simulink model "L3Pilot_AEB_v1"  (R2021b)
settings: Solver=FixedStepAuto  StartTime=0.0  StopTime=350  RelTol=1e-3  EnableMultiTasking=on
values from neighbouring files (symbols this model uses):
  t_takeover = 70    [Var_L3Pilot_ADF_v1.m]
  Tabt = 0.1    [Var_L3Pilot_ADF_v1.m]
undefined symbols (not defined in the file or in its folder): ComponentState
libraries: simulink x2
settings Model: Creator=QXV8396  LastModifiedBy=Q395473
settings SolverCC: AlgebraicLoopSolver=TrustRegion
settings DataIOCC: LimitDataPoints=on  ReturnWorkspaceOutputs=off
settings DebuggingCC: AllowSymbolicDim=off  SFUnexpectedBacktrackingDiag=warning  SFNoUnconditionalDefaultTransitionDiag=warning  SFExecutionAtInitializationDiag=none  SFMachineParentedDataDiag=warning  ArithmeticOperatorsInVariantConditions=warning
settings ModelReferenceCC: PropagateSignalLabelsOutOfModel=off
settings SFSimCC: SimUseLocalCustomCode=off  CustomCodeUndefinedFunction=UseInterfaceOnly
settings RTWCC: Description=FMU Co-Simulation 1.0 Standalone  SystemTargetFile=fmu_cs1.tlc  MakeCommand=make_rtw FMIT_INTERMEDIATE_LIB_DIR=DEFAULT FMIT_ADDITIONAL_CFLAGS=  TemplateMakefile=fmu_cs1_default_tmf  RTWUseLocalCustomCode=off
settings CodeAppCC: StateflowObjectComments=on
settings STFCustomTargetCC: MATLABClassNameForMDSCustomization=Simulink.SoftwareTarget.TargetSpecificTriggerConfigurationBase  SystemTargetFile=fmu_cs1.tlc
settings ConfigComp: CovMetricSettings=dw  CovSaveCumulativeToWorkspaceVar=on  CovSaveSingleToWorkspaceVar=on  CovExternalEMLEnable=off

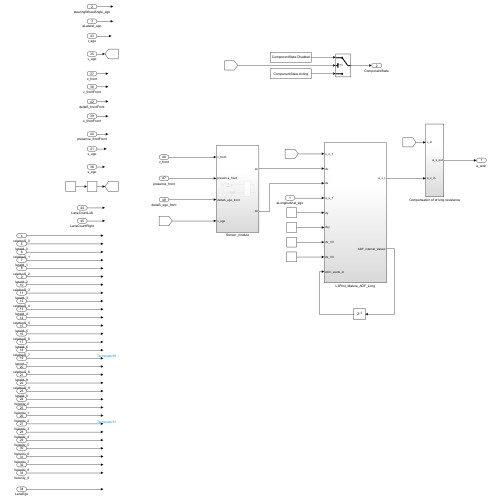
[thumbnail: Simulink's stored preview of the top-level diagram]
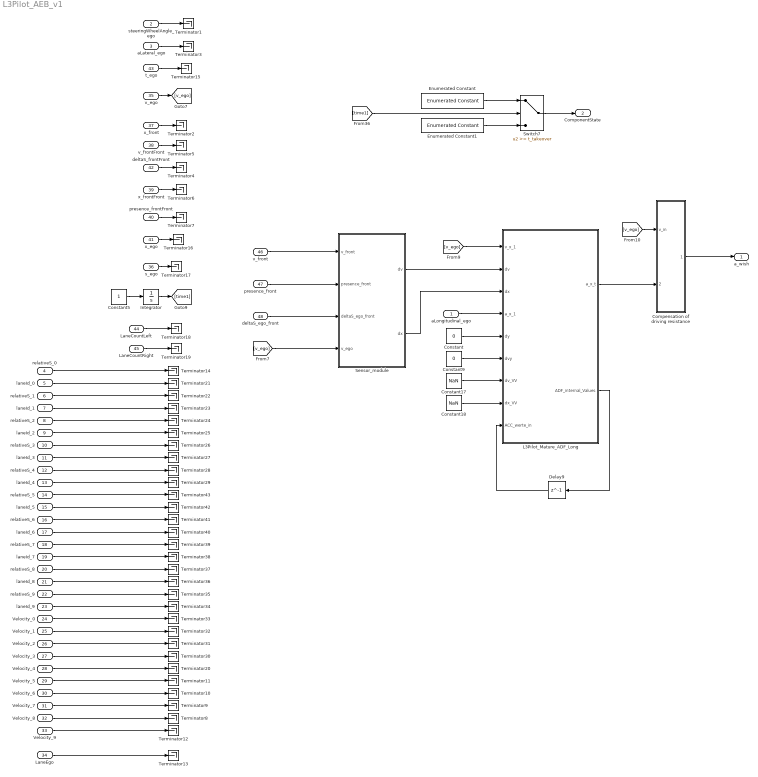
== system L3Pilot_AEB_v1 ==
  aLongitudinal_ego : Inport
  steeringWheelAngle_ego : Inport  Port=2
  aLateral_ego : Inport  Port=3
  relativeS_0 : Inport  Port=4  OutDataTypeStr=double
  laneId_0 : Inport  Port=5  OutDataTypeStr=int8
  relativeS_1 : Inport  Port=6  OutDataTypeStr=double
  laneId_1 : Inport  Port=7  OutDataTypeStr=int8
  relativeS_2 : Inport  Port=8  OutDataTypeStr=double
  laneId_2 : Inport  Port=9  OutDataTypeStr=int8
  relativeS_3 : Inport  Port=10  OutDataTypeStr=double
  laneId_3 : Inport  Port=11  OutDataTypeStr=int8
  relativeS_4 : Inport  Port=12  OutDataTypeStr=double
  laneId_4 : Inport  Port=13  OutDataTypeStr=int8
  relativeS_5 : Inport  Port=14  OutDataTypeStr=double
  laneId_5 : Inport  Port=15  OutDataTypeStr=int8
  relativeS_6 : Inport  Port=16  OutDataTypeStr=double
  laneId_6 : Inport  Port=17  OutDataTypeStr=int8
  relativeS_7 : Inport  Port=18  OutDataTypeStr=double
  laneId_7 : Inport  Port=19  OutDataTypeStr=int8
  relativeS_8 : Inport  Port=20  OutDataTypeStr=double
  laneId_8 : Inport  Port=21  OutDataTypeStr=int8
  relativeS_9 : Inport  Port=22  OutDataTypeStr=double
  laneId_9 : Inport  Port=23  OutDataTypeStr=int8
  Velocity_0 : Inport  Port=24  OutDataTypeStr=double
  Velocity_1 : Inport  Port=25  OutDataTypeStr=double
  Velocity_2 : Inport  Port=26  OutDataTypeStr=double
  Velocity_3 : Inport  Port=27  OutDataTypeStr=double
  Velocity_4 : Inport  Port=28  OutDataTypeStr=double
  Velocity_5 : Inport  Port=29  OutDataTypeStr=double
  Velocity_6 : Inport  Port=30  OutDataTypeStr=double
  Velocity_7 : Inport  Port=31  OutDataTypeStr=double
  Velocity_8 : Inport  Port=32  OutDataTypeStr=double
  Velocity_9 : Inport  Port=33  OutDataTypeStr=double
  LaneEgo : Inport  Port=34  OutDataTypeStr=int8
  v_ego : Inport  Port=35  OutDataTypeStr=double
  s_ego : Inport  Port=36
  x_front : Inport  Port=37  OutDataTypeStr=double
  v_frontFront : Inport  Port=38  OutDataTypeStr=double
  x_frontFront : Inport  Port=39  OutDataTypeStr=double
  presence_frontFront : Inport  Port=40  OutDataTypeStr=boolean
  x_ego : Inport  Port=41
  deltaS_frontFront : Inport  Port=42  OutDataTypeStr=double
  t_ego : Inport  Port=43
  LaneCountLeft : Inport  Port=44  OutDataTypeStr=int8
  LaneCountRight : Inport  Port=45  OutDataTypeStr=int8
  v_front : Inport  Port=46  OutDataTypeStr=double
  presence_front : Inport  Port=47  OutDataTypeStr=boolean
  deltaS_ego_front : Inport  Port=48
  Compensation of driving resistance : Subsystem
  Constant : Constant  Value=0  SampleTime=Tabt
  Constant17 : Constant  Value=NaN  SampleTime=Tabt
  Constant18 : Constant  Value=NaN  SampleTime=Tabt
  Constant5 : Constant  SampleTime=Tabt
  Constant9 : Constant  Value=0  SampleTime=Tabt
  Delay9 : Delay  DelayLength=1  InitialCondition=0  SampleTime=Tabt
  Enumerated Constant : simulink/Sources/Enumerated Constant  OutDataTypeStr=Enum: ComponentState  Value=ComponentState.Disabled  SampleTime=inf
  Enumerated Constant1 : simulink/Sources/Enumerated Constant  OutDataTypeStr=Enum: ComponentState  Value=ComponentState.Acting  SampleTime=inf
  Integrator : Integrator
  L3Pilot_Mature_ADF_Long : Subsystem
  Sensor_module : Subsystem
  Switch7 : Switch  Threshold=t_takeover
  Terminator{1..43} (43 alike) : Terminator
  a_wish : Outport  VectorParamsAs1DForOutWhenUnconnected=off
  ComponentState : Outport  Port=2  OutDataTypeStr=Enum: ComponentState  VectorParamsAs1DForOutWhenUnconnected=off
  wires:
  Constant17/1 -> L3Pilot_Mature_ADF_Long/7(dv_VV)
  Constant18/1 -> L3Pilot_Mature_ADF_Long/8(dx_VV)
  Constant9/1 -> L3Pilot_Mature_ADF_Long/6(dvy)
  Constant/1 -> L3Pilot_Mature_ADF_Long/5(dy)
  Delay9/1 -> L3Pilot_Mature_ADF_Long/9(ACC_werte_in)
  aLongitudinal_ego/1 -> L3Pilot_Mature_ADF_Long/4("a_x_1 ")
  L3Pilot_Mature_ADF_Long/2(ADF_internal_Values) -> Delay9/1
  [v_ego] -> L3Pilot_Mature_ADF_Long/1(v_x_1)
  [v_ego] -> Compensation of driving resistance/1(v_in)
  Sensor_module/1(dv) -> L3Pilot_Mature_ADF_Long/2(dv)
  Sensor_module/2(dx) -> L3Pilot_Mature_ADF_Long/3(dx)
  L3Pilot_Mature_ADF_Long/1(a_x_t) -> Compensation of driving resistance/2(a_x_in)
  Compensation of driving resistance/1(a_x_out) -> a_wish/1
  relativeS_1/1 -> Terminator22/1
  Velocity_2/1 -> Terminator31/1
  laneId_9/1 -> Terminator34/1
  relativeS_4/1 -> Terminator28/1
  [time1] -> Switch7/2
  Velocity_4/1 -> Terminator20/1
  Switch7/1 -> ComponentState/1
  Velocity_8/1 -> Terminator8/1
  Velocity_9/1 -> Terminator12/1
  relativeS_8/1 -> Terminator37/1
  relativeS_2/1 -> Terminator24/1
  relativeS_9/1 -> Terminator35/1
  Velocity_1/1 -> Terminator32/1
  relativeS_7/1 -> Terminator39/1
  relativeS_6/1 -> Terminator41/1
  relativeS_0/1 -> Terminator14/1
  laneId_7/1 -> Terminator38/1
  relativeS_5/1 -> Terminator43/1
  laneId_2/1 -> Terminator25/1
  laneId_3/1 -> Terminator27/1
  laneId_1/1 -> Terminator23/1
  Velocity_3/1 -> Terminator30/1
  Velocity_6/1 -> Terminator10/1
  LaneEgo/1 -> Terminator13/1
  Velocity_7/1 -> Terminator9/1
  Velocity_5/1 -> Terminator11/1
  relativeS_3/1 -> Terminator26/1
  laneId_6/1 -> Terminator40/1
  laneId_8/1 -> Terminator36/1
  laneId_4/1 -> Terminator29/1
  Enumerated Constant1/1 -> Switch7/3
  Enumerated Constant/1 -> Switch7/1
  laneId_5/1 -> Terminator42/1
  laneId_0/1 -> Terminator21/1
  Velocity_0/1 -> Terminator33/1
  x_front/1 -> Terminator2/1
  t_ego/1 -> Terminator15/1
  x_frontFront/1 -> Terminator6/1
  x_ego/1 -> Terminator16/1
  Integrator/1 -> [time1]
  s_ego/1 -> Terminator17/1
  Constant5/1 -> Integrator/1
  deltaS_frontFront/1 -> Terminator4/1
  LaneCountLeft/1 -> Terminator18/1
  LaneCountRight/1 -> Terminator19/1
  v_frontFront/1 -> Terminator5/1
  v_ego/1 -> [v_ego]
  presence_frontFront/1 -> Terminator7/1
  v_front/1 -> Sensor_module/1(v_front)
  [v_ego] -> Sensor_module/4(v_ego)
  presence_front/1 -> Sensor_module/2(presence_front)
  deltaS_ego_front/1 -> Sensor_module/3(deltaS_ego_front)
  steeringWheelAngle_ego/1 -> Terminator1/1
  aLateral_ego/1 -> Terminator3/1

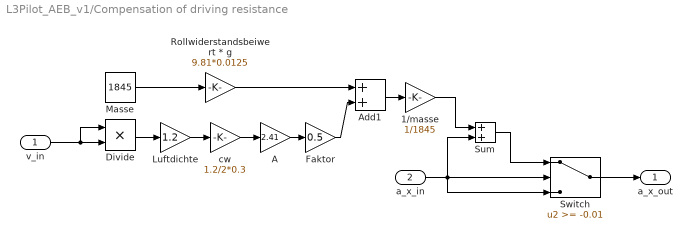
== system L3Pilot_AEB_v1/Compensation of driving resistance ==
  v_in : Inport
  a_x_in : Inport  Port=2
  1/masse : Gain  Gain=1/1845
  A : Gain  Gain=2.41  OutDataTypeStr=double
  Add1 : Sum
  Divide : Product  Inputs=**
  Faktor : Gain  Gain=0.5  OutDataTypeStr=double
  Luftdichte : Gain  Gain=1.2  OutDataTypeStr=double
  Masse : Constant  Value=1845
  Rollwiderstandsbeiwert * g : Gain  Gain=9.81*0.0125
  Sum : Sum
  Switch : Switch  Threshold=-0.01
  cw : Gain  Gain=1.2/2*0.3  OutDataTypeStr=double
  a_x_out : Outport  VectorParamsAs1DForOutWhenUnconnected=off
  wires:
  Divide/1 -> Luftdichte/1
  Add1/1 -> 1/masse/1
  a_x_in/1 -> Sum/2, Switch/3, Switch/2
  Switch/1 -> a_x_out/1
  Masse/1 -> Rollwiderstandsbeiwert * g/1
  v_in/1 -> Divide/1, Divide/2
  1/masse/1 -> Sum/1
  Sum/1 -> Switch/1
  Rollwiderstandsbeiwert * g/1 -> Add1/1
  cw/1 -> A/1
  Luftdichte/1 -> cw/1
  A/1 -> Faktor/1
  Faktor/1 -> Add1/2

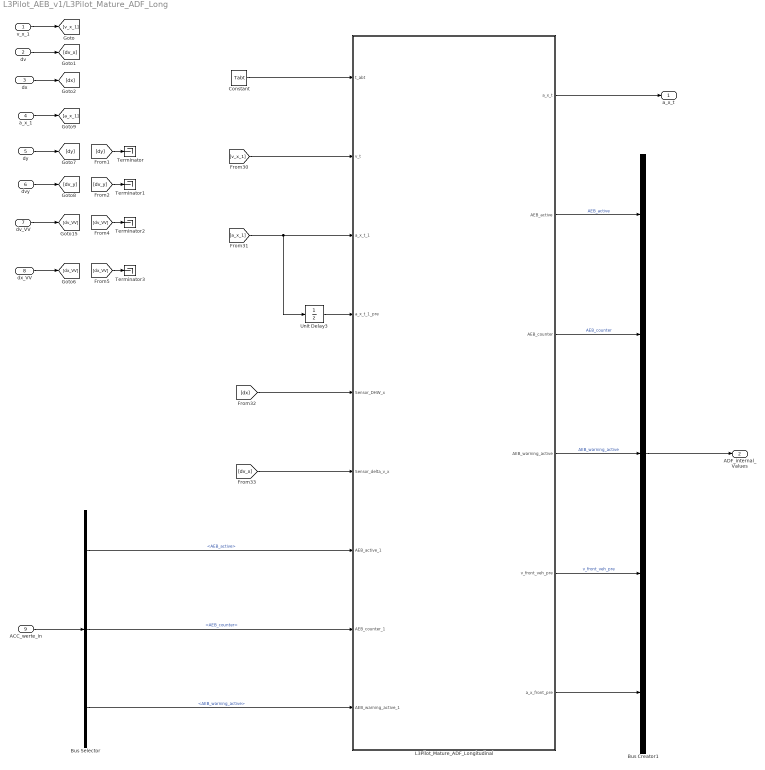
== system L3Pilot_AEB_v1/L3Pilot_Mature_ADF_Long ==
  v_x_1 : Inport
  dv : Inport  Port=2
  dx : Inport  Port=3
  "a_x_1 " : Inport  Port=4
  dy : Inport  Port=5
  dvy : Inport  Port=6
  dv_VV : Inport  Port=7
  dx_VV : Inport  Port=8
  ACC_werte_in : Inport  Port=9
  Bus Creator1 : BusCreator  Inputs=5
  Bus Selector : BusSelector  OutputSignals=AEB_active,AEB_counter,AEB_warning_active
  Constant : Constant  Value=Tabt
  L3Pilot_Mature_ADF_Longitudinal : MATLAB Function  TreatAsAtomicUnit=on
  Terminator{,1..3} (4 alike) : Terminator
  Unit Delay3 : UnitDelay  SampleTime=-1  HasFrameUpgradeWarning=on
  a_x_t : Outport  VectorParamsAs1DForOutWhenUnconnected=off
  ADF_internal_Values : Outport  Port=2  VectorParamsAs1DForOutWhenUnconnected=off
  wires:
  v_x_1/1 -> [v_x_1]
  dv/1 -> [dv_x]
  dx/1 -> [dx]
  dy/1 -> [dy]
  dvy/1 -> [dv_y]
  "a_x_1 "/1 -> [a_x_1]
  Bus Creator1/1 -> ADF_internal_Values/1
  ACC_werte_in/1 -> Bus Selector/1
  Constant/1 -> L3Pilot_Mature_ADF_Longitudinal/1(t_abt)
  [v_x_1] -> L3Pilot_Mature_ADF_Longitudinal/2(v_t)
  [a_x_1] -> Unit Delay3/1, L3Pilot_Mature_ADF_Longitudinal/3(a_x_t_1)
  L3Pilot_Mature_ADF_Longitudinal/1(a_x_t) -> a_x_t/1
  [dx] -> L3Pilot_Mature_ADF_Longitudinal/5(Sensor_DHW_x)
  [dv_x] -> L3Pilot_Mature_ADF_Longitudinal/6(Sensor_delta_v_x)
  dx_VV/1 -> [dx_VV]
  dv_VV/1 -> [dv_VV]
  [dy] -> Terminator/1
  [dv_y] -> Terminator1/1
  L3Pilot_Mature_ADF_Longitudinal/2(AEB_active) -> Bus Creator1/1  "AEB_active"
  L3Pilot_Mature_ADF_Longitudinal/3(AEB_counter) -> Bus Creator1/2  "AEB_counter"
  Bus Selector/1 -> L3Pilot_Mature_ADF_Longitudinal/7(AEB_active_1)  "<AEB_active>"
  Bus Selector/2 -> L3Pilot_Mature_ADF_Longitudinal/8(AEB_counter_1)  "<AEB_counter>"
  Unit Delay3/1 -> L3Pilot_Mature_ADF_Longitudinal/4(a_x_t_1_pre)
  L3Pilot_Mature_ADF_Longitudinal/4(AEB_warning_active) -> Bus Creator1/3  "AEB_warning_active"
  Bus Selector/3 -> L3Pilot_Mature_ADF_Longitudinal/9(AEB_warning_active_1)  "<AEB_warning_active>"
  [dv_VV] -> Terminator2/1
  [dx_VV] -> Terminator3/1
  L3Pilot_Mature_ADF_Longitudinal/5(v_front_veh_pre) -> Bus Creator1/4  "v_front_veh_pre"
  L3Pilot_Mature_ADF_Longitudinal/6(a_x_front_pre) -> Bus Creator1/5

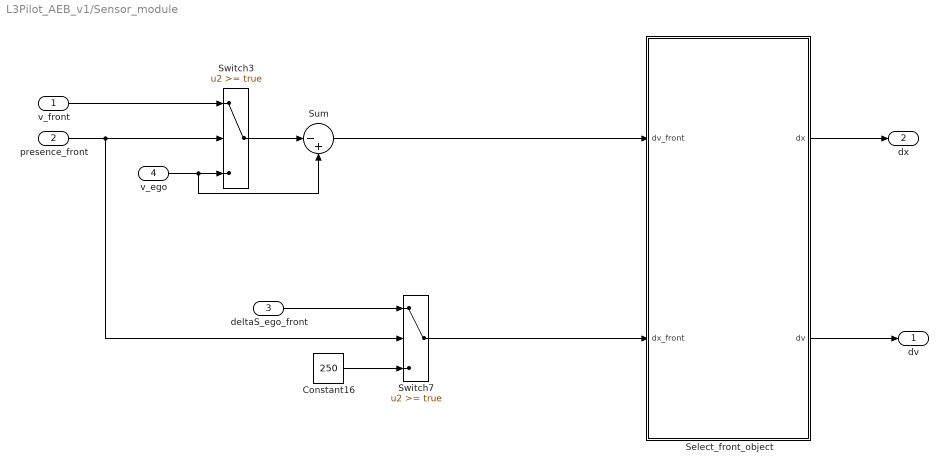
== system L3Pilot_AEB_v1/Sensor_module ==
  v_front : Inport
  presence_front : Inport  Port=2  OutDataTypeStr=boolean
  deltaS_ego_front : Inport  Port=3
  v_ego : Inport  Port=4  OutDataTypeStr=double
  Constant16 : Constant  Value=250  SampleTime=Tabt
  Select_front_object : MATLAB Function  TreatAsAtomicUnit=on
  Sum : Sum  Inputs=|-+
  Switch3 : Switch  Threshold=true
  Switch7 : Switch  Threshold=true
  dv : Outport  VectorParamsAs1DForOutWhenUnconnected=off
  dx : Outport  Port=2  VectorParamsAs1DForOutWhenUnconnected=off
  wires:
  v_front/1 -> Switch3/1
  Switch3/1 -> Sum/1
  Sum/1 -> Select_front_object/1(dv_front)
  deltaS_ego_front/1 -> Switch7/1
  presence_front/1 -> Switch7/2, Switch3/2
  Constant16/1 -> Switch7/3
  v_ego/1 -> Sum/2, Switch3/3
  Switch7/1 -> Select_front_object/2(dx_front)
  Select_front_object/1(dx) -> dx/1
  Select_front_object/2(dv) -> dv/1

== matlab function L3Pilot_AEB_v1/L3Pilot_Mature_ADF_Long/L3Pilot_Mature_ADF_Longitudinal ==
  data: t_abt input; v_t input; a_x_t_1 input; a_x_t_1_pre input; a_x_t output; Sensor_DHW_x input; Sensor_delta_v_x input; AEB_active_1 input; AEB_counter_1 input; AEB_warning_active_1 input; AEB_active output; AEB_counter output; AEB_warning_active output; v_front_veh_pre output; a_x_front_pre output
function [a_x_t,AEB_active,AEB_counter,AEB_warning_active,v_front_veh_pre,a_x_front_pre]  =L3Pilot_Mature_AEB...
    (t_abt,v_t,a_x_t_1,a_x_t_1_pre,Sensor_DHW_x,Sensor_delta_v_x,AEB_active_1,AEB_counter_1,AEB_warning_active_1)

%%%%%%%%%%%%%%%%%%%%%%%%%%%%%%%%%%%%%%%%%%%%%%%%%%%%%%%%%%%%%%%%%%%%%%%%%%%
v_current = v_t;

Obj_x = Sensor_DHW_x-2;

dv_current = Sensor_delta_v_x;

v_front_veh = v_current-dv_current;

%%%%%%%%%%%%%%%%%%%%%%%%%%%%%%%%%%%%%%%%%%%%%%%%%%%%%%%%%%%%%%%%%%%%%%%%%%%

%%%%%%%%%%%%%%%%%%%%%%%%%%%%%%%%%%%%%%%%%%%%%%%%%%%%%%%%%%%%%%%%%%%%%%%%%%%
% AEB Parameters

t_brake_stage_1 = 0.4;
a_x_build_up_velocity_1 = 35;
a_x_build_up_velocity_2 = 35;

if dv_current>0 && Obj_x<200 
    TTC_front = Obj_x./dv_current;
else
    TTC_front =999;
end

x_remain = 0.5;
if dv_current >-0.5
    a_required = min([a_x_t_1_pre,-(dv_current.^2) / (2 * (Obj_x-x_remain))]);
else
    a_required = -1;
end

v_AEB = [0,10,20,30,40,50,60,70,80,90,100,110,120,130,140,150,250]/3.6;
threshold_AEB_warning = [1.2 1.2 1.3 1.4 1.5 1.6 1.7 1.8 1.9 1.9 1.9 1.9 1.9 1.9 1.9 1.9 1.9];

if v_front_veh>1
    % Front vehicle Moving
    threshold_AEB = [0.85 0.85 0.9 0.95 1.1 1.2 1.3 1.4 1.5 1.5 1.5 1.5 1.5 1.5 1.5 1.5 1.5 ];
else
    % Front vehicle stand still
    threshold_AEB = [0.75 0.75 0.8 0.95 1.1 1.2 1.4 1.4 1.4 1.4 1.4 1.4 1.4 1.4 1.4 1.4 1.4];
end

current_threshold_warning = interp1(v_AEB,threshold_AEB_warning,v_current);
current_threshold = interp1(v_AEB,threshold_AEB,v_current);


%%%%%%%%%%%%%%%%%%%%%%%%%%%%%%%%%%%%%%%%%%%%%%%%%%%%%%%%%%%%%%%%%%%%%%%%%%%
% AEB Warning
if TTC_front<current_threshold_warning
    AEB_warning_active = 1;
else
    if a_required>=0 && AEB_warning_active_1==1
        AEB_warning_active = 1;
    else
        AEB_warning_active = 0;
    end
end

%%%%%%%%%%%%%%%%%%%%%%%%%%%%%%%%%%%%%%%%%%%%%%%%%%%%%%%%%%%%%%%%%%%%%%%%%%%
% AEB Control

if TTC_front<current_threshold
   AEB_active = 1;
   AEB_counter = AEB_counter_1+t_abt;
else
   if AEB_active_1 ==1 && a_required>1
        AEB_active = 1;
        AEB_counter = AEB_counter_1+t_abt;
   else
        AEB_active =0;
        AEB_counter = 0;
   end
end

if AEB_active_1 ==1
    if AEB_counter<= t_brake_stage_1
        a_AEB_brake = max([a_x_t_1_pre-a_x_build_up_velocity_1*t_abt,-3.5]);        
    else
        a_AEB_brake = max([a_x_t_1_pre-a_x_build_up_velocity_2*t_abt,a_required,-9.81]);
    end   
else
    a_AEB_brake = NaN;
end

%%%%%%%%%%%%%%%%%%%%%%%%%%%%%%%%%%%%%%%%%%%%%%%%%%%%%%%%%%%%%%%%%%%%%%%%%%%
% Longitudinal Control

a_x_t = nanmin([a_x_t_1,a_AEB_brake]);

v_front_veh_pre = v_front_veh;
a_x_front_pre = a_x_front_PT1;

== matlab function L3Pilot_AEB_v1/Sensor_module/Select_front_object ==
  data: dv_front input; dx output; dx_front input; dv output
function [dx,dv] = Select_front_object(dv_front,   dx_front)



dx = dx_front;
dv = dv_front;
